simulink model "Project2_400100792"  (R2021b)
settings: Solver=ode23t  StartTime=0.0  StopTime=25  FixedStep=0.01  MaxStep=0.001  RelTol=1e-3
values from neighbouring files (symbols this model uses):
  g = 9.8    [parameters.m]
  Jw = 0.01    [parameters.m]
  K = 1000    [parameters.m]
  mv = 1400    [parameters.m]
  roadType = 4    [Q2.m]    (also in parameters.m = 1)
  rw = 0.32    [parameters.m]
  T = 0.05    [parameters.m]
  Tbmax = 2000    [parameters.m]
  v0 = 33.33    [parameters.m]
  vmin = 1.5    [parameters.m]
settings Model: Creator=baten  LastModifiedBy=baten

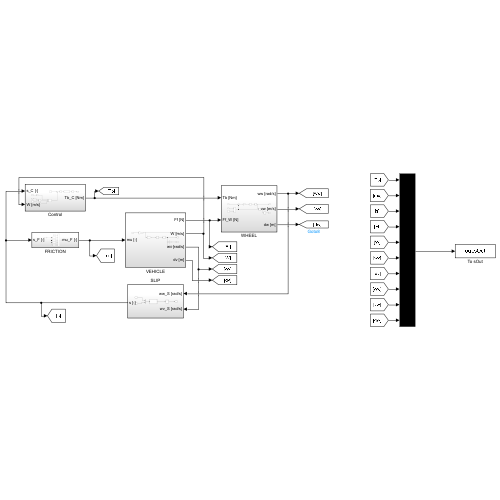
[thumbnail: Simulink's stored preview of the top-level diagram]
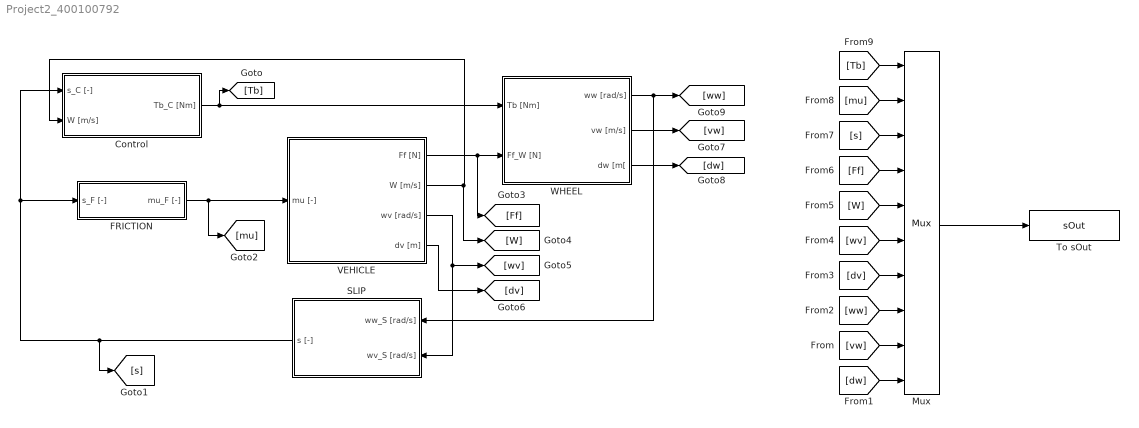
== system Project2_400100792 ==
  Control : Subsystem
  FRICTION : Subsystem
  Mux : Mux  Inputs=10
  SLIP : Subsystem
  To sOut : ToWorkspace  VariableName=sOut  SampleTime=-1
  VEHICLE : Subsystem
  WHEEL : Subsystem
  wires:
  SLIP/1(s [-]) -> [s], FRICTION/1(s_F [-]), Control/1(s_C [-])
  VEHICLE/2(W [m/s]) -> [W], Control/2(W [m/s])
  Control/1(Tb_C [Nm]) -> [Tb], WHEEL/1(Tb [Nm])
  VEHICLE/1(Ff [N]) -> [Ff], WHEEL/2(Ff_W [N])
  VEHICLE/3(wv [rad/s]) -> [wv], SLIP/2(wv_S [rad/s])
  WHEEL/1(ww [rad/s]) -> SLIP/1(ww_S [rad/s]), [ww]
  FRICTION/1(mu_F [-]) -> [mu], VEHICLE/1(mu [-])
  Mux/1 -> To sOut/1
  [Tb] -> Mux/1
  [mu] -> Mux/2
  [s] -> Mux/3
  [Ff] -> Mux/4
  [dv] -> Mux/7
  [dw] -> Mux/10
  [vw] -> Mux/9
  [ww] -> Mux/8
  [wv] -> Mux/6
  [W] -> Mux/5
  WHEEL/2(vw [m/s]) -> [vw]
  WHEEL/3(dw [m[) -> [dw]
  VEHICLE/4(dv [m]) -> [dv]

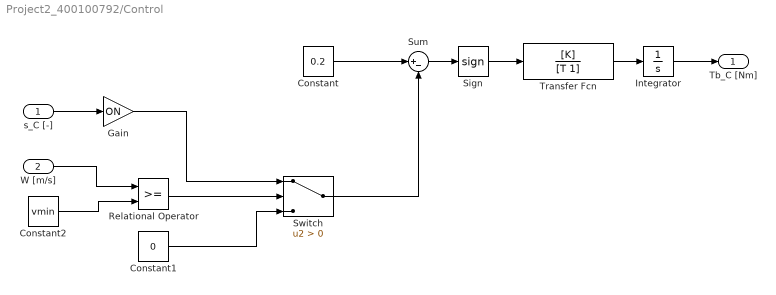
== system Project2_400100792/Control ==
  s_C [-] : Inport
  W [m/s] : Inport  Port=2
  Constant : Constant  Value=0.2
  Constant1 : Constant  Value=0
  Constant2 : Constant  Value=vmin
  Gain : Gain  Gain=ON
  Integrator : Integrator  LimitOutput=on  UpperSaturationLimit=Tbmax  LowerSaturationLimit=0
  Relational Operator : RelationalOperator  OutDataTypeStr=boolean  RndMeth=Simplest
  Sign : Signum
  Sum : Sum  Inputs=|+-
  Switch : Switch  Criteria=u2 > Threshold
  Transfer Fcn : TransferFcn  Numerator=[K]  Denominator=[T 1]
  Tb_C [Nm] : Outport
  wires:
  Sum/1 -> Sign/1
  Constant1/1 -> Switch/3
  Relational Operator/1 -> Switch/2
  Switch/1 -> Sum/2
  Sign/1 -> Transfer Fcn/1
  Integrator/1 -> Tb_C [Nm]/1
  s_C [-]/1 -> Gain/1
  W [m/s]/1 -> Relational Operator/1
  Transfer Fcn/1 -> Integrator/1
  Constant2/1 -> Relational Operator/2
  Gain/1 -> Switch/1
  Constant/1 -> Sum/1

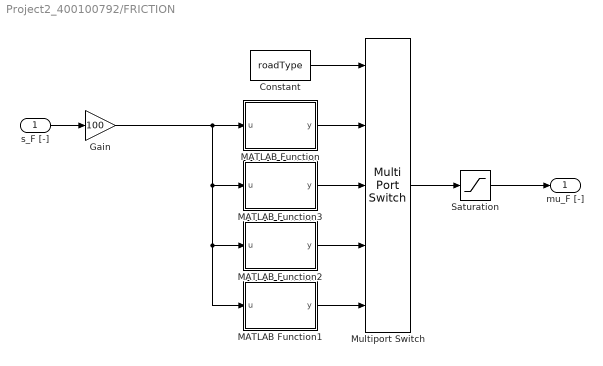
== system Project2_400100792/FRICTION ==
  s_F [-] : Inport
  Constant : Constant  Value=roadType
  Gain : Gain  Gain=100
  MATLAB Function : MATLAB Function  TreatAsAtomicUnit=on
  MATLAB Function1 : MATLAB Function  TreatAsAtomicUnit=on
  MATLAB Function2 : MATLAB Function  TreatAsAtomicUnit=on
  MATLAB Function3 : MATLAB Function  TreatAsAtomicUnit=on
  Multiport Switch : MultiPortSwitch  Inputs=4
  Saturation : Saturate  UpperLimit=1  LowerLimit=0
  mu_F [-] : Outport
  wires:
  Gain/1 -> MATLAB Function/1(u), MATLAB Function3/1(u), MATLAB Function2/1(u), MATLAB Function1/1(u)
  s_F [-]/1 -> Gain/1
  Constant/1 -> Multiport Switch/1
  Multiport Switch/1 -> Saturation/1
  Saturation/1 -> mu_F [-]/1
  MATLAB Function/1(y) -> Multiport Switch/2
  MATLAB Function3/1(y) -> Multiport Switch/3
  MATLAB Function2/1(y) -> Multiport Switch/4
  MATLAB Function1/1(y) -> Multiport Switch/5

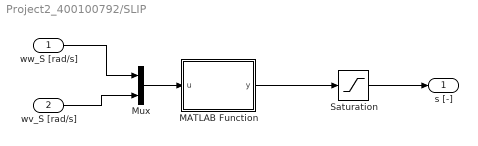
== system Project2_400100792/SLIP ==
  ww_S [rad/s] : Inport
  wv_S [rad/s] : Inport  Port=2
  MATLAB Function : MATLAB Function  TreatAsAtomicUnit=on
  Mux : Mux  Inputs=2
  Saturation : Saturate  UpperLimit=1  LowerLimit=0
  s [-] : Outport
  wires:
  Saturation/1 -> s [-]/1
  MATLAB Function/1(y) -> Saturation/1
  Mux/1 -> MATLAB Function/1(u)
  ww_S [rad/s]/1 -> Mux/1
  wv_S [rad/s]/1 -> Mux/2

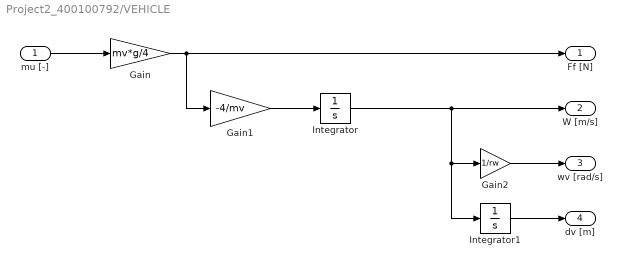
== system Project2_400100792/VEHICLE ==
  mu [-] : Inport
  Gain : Gain  Gain=mv*g/4
  Gain1 : Gain  Gain=-4/mv
  Gain2 : Gain  Gain=1/rw
  Integrator : Integrator  InitialCondition=v0  LimitOutput=on  UpperSaturationLimit=1000  LowerSaturationLimit=0.001
  Integrator1 : Integrator
  Ff [N] : Outport
  W [m/s] : Outport  Port=2
  wv [rad/s] : Outport  Port=3
  dv [m] : Outport  Port=4
  wires:
  Gain/1 -> Ff [N]/1, Gain1/1
  Integrator/1 -> W [m/s]/1, Integrator1/1, Gain2/1
  Integrator1/1 -> dv [m]/1
  Gain1/1 -> Integrator/1
  Gain2/1 -> wv [rad/s]/1
  mu [-]/1 -> Gain/1

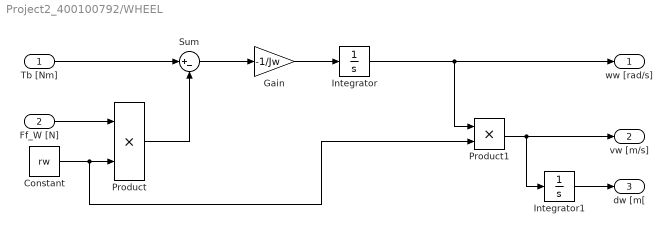
== system Project2_400100792/WHEEL ==
  Tb [Nm] : Inport
  Ff_W [N] : Inport  Port=2
  Constant : Constant  Value=rw
  Gain : Gain  Gain=-1/Jw
  Integrator : Integrator  InitialCondition=v0/rw  LimitOutput=on  UpperSaturationLimit=1000  LowerSaturationLimit=0
  Integrator1 : Integrator
  Product : Product
  Product1 : Product
  Sum : Sum  Inputs=|+-
  ww [rad/s] : Outport
  vw [m/s] : Outport  Port=2
  dw [m[ : Outport  Port=3
  wires:
  Product1/1 -> vw [m/s]/1, Integrator1/1
  Product/1 -> Sum/2
  Integrator/1 -> ww [rad/s]/1, Product1/1
  Integrator1/1 -> dw [m[/1
  Constant/1 -> Product1/2, Product/2
  Gain/1 -> Integrator/1
  Sum/1 -> Gain/1
  Ff_W [N]/1 -> Product/1
  Tb [Nm]/1 -> Sum/1

== matlab function Project2_400100792/SLIP/MATLAB Function ==
  data: u input; y output
function y = fcn(u)
    y = 1 - u(1)/(u(2) + (u(2)==0)*eps);
end

== matlab function Project2_400100792/FRICTION/MATLAB Function1 ==
  data: u input; y output
function y = fcn(u)

y = 0.1*(1.07*(1-exp(-0.38*u))-0.007*u);

== matlab function Project2_400100792/FRICTION/MATLAB Function2 ==
  data: u input; y output
function y = fcn(u)

y = 0.3*(1.07*(1-exp(-0.1773*u))-0.006*u);

== matlab function Project2_400100792/FRICTION/MATLAB Function3 ==
  data: u input; y output
function y = fcn(u)

y = 0.7*(1.07*(1-exp(-0.5*u))-0.003*u);

== matlab function Project2_400100792/FRICTION/MATLAB Function ==
  data: u input; y output
function y = fcn(u)

y = 0.9*(1.07*(1-exp(-0.2773*u))-0.0026*u);
